simulink model "ode_simulation"  (R2022a)
settings: Solver=VariableStepAuto  StartTime=0.0  StopTime=60  RelTol=1e-3
libraries: slident x2
settings Model: Creator=mjwhi  LastModifiedBy=mjsung2

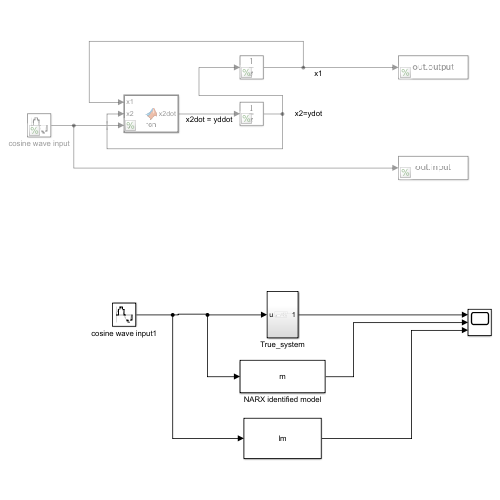
[thumbnail: Simulink's stored preview of the top-level diagram]
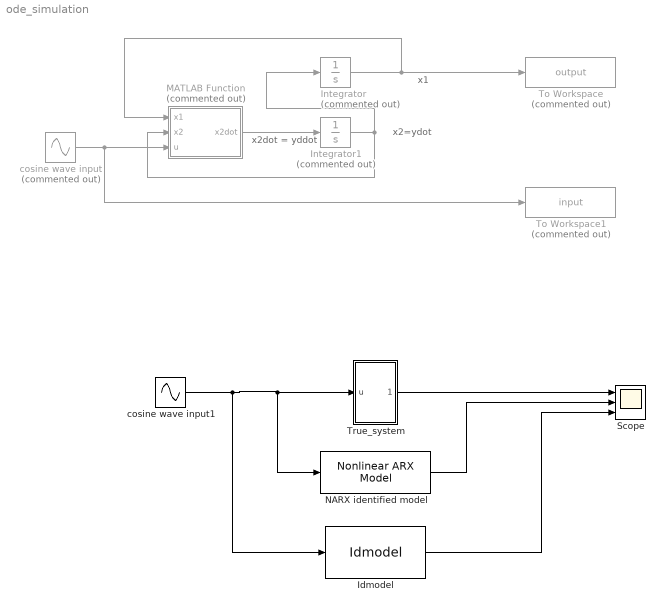
== system ode_simulation ==
  note: x1
  note: x2dot = yddot
  note: x2=ydot
  Idmodel : slident/Models/Idmodel  sys=lm  IC=0  noi=on  seed=[]
      settings: SourceProductBaseCode=ID
  Integrator : Integrator  Commented=on
  Integrator1 : Integrator  Commented=on
  MATLAB Function : MATLAB Function  Commented=on  TreatAsAtomicUnit=on
  NARX identified model : slident/Models/Nonlinear ARX Model  sys=m  ICspec=Input and output values  X0=0  U0=0  Y0=0
      settings: SourceProductBaseCode=ID
  Scope : Scope  NumInputPorts=3
  To Workspace : ToWorkspace  Commented=on  VariableName=output  SaveFormat=Timeseries  SampleTime=0.02
  To Workspace1 : ToWorkspace  Commented=on  VariableName=input  SaveFormat=Timeseries  SampleTime=0.02
  True_system : Subsystem
  cosine wave input : Sin  Commented=on  Amplitude=37  Phase=pi/2  SampleTime=0.02
  cosine wave input1 : Sin  Amplitude=37  Phase=pi/2  SampleTime=0.02
  wires:
  Integrator/1 -> MATLAB Function/1(x1), To Workspace/1
  Integrator1/1 -> MATLAB Function/2(x2), Integrator/1
  cosine wave input/1 -> To Workspace1/1, MATLAB Function/3(u)
  MATLAB Function/1(x2dot) -> Integrator1/1
  True_system/1(Out1) -> Scope/1
  NARX identified model/1 -> Scope/2
  cosine wave input1/1 -> Idmodel/1, NARX identified model/1, True_system/1(u)
  Idmodel/1 -> Scope/3

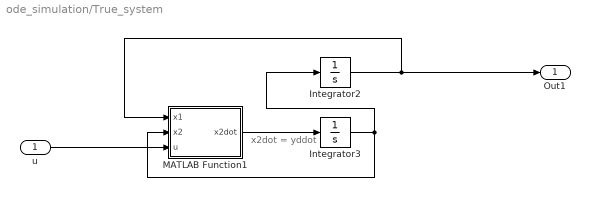
== system ode_simulation/True_system ==
  note: x2dot = yddot
  u : Inport
  Integrator2 : Integrator
  Integrator3 : Integrator
  MATLAB Function1 : MATLAB Function  TreatAsAtomicUnit=on
  Out1 : Outport
  wires:
  Integrator3/1 -> MATLAB Function1/2(x2), Integrator2/1
  Integrator2/1 -> Out1/1, MATLAB Function1/1(x1)
  MATLAB Function1/1(x2dot) -> Integrator3/1
  u/1 -> MATLAB Function1/3(u)

== matlab function ode_simulation/MATLAB Function ==
  data: x1 input; x2 input; u input; x2dot output
function x2dot = fcn(x1, x2, u)
a= 0.1;
b=-0.5;
c=0.5;
x2dot = -a*(x1^2-1)/(x1^2+1)*x2-b*x1-c*x1^3+u;

== matlab function ode_simulation/True_system/MATLAB Function1 ==
  data: x1 input; x2 input; u input; x2dot output
function x2dot = fcn(x1, x2, u)
a= 0.1;
b=-0.5;
c=0.5;
x2dot = -a*(x1^2-1)/(x1^2+1)*x2-b*x1-c*x1^3+u;
